simulink model "quest3"  (R2015a)
settings: Solver=ode5  StartTime=0.0  StopTime=20  FixedStep=0.001  RelTol=1e-3
values from neighbouring files (symbols this model uses):
  a = 0.3    [dynamicInit.m]
  a_e = a    (= 0.3)    [dynamicInit.m]
  d = 0.1    [dynamicInit.m]    (also in plotVehicle.m)
  r = 0.1    [dynamicInit.m]
  r_e = r    (= 0.1)    [dynamicInit.m]
undefined symbols (not defined in the file or in its folder): F_invW_1
libraries: simulink x2
settings Model: CovModelRefEnable=off  Creator=Subodh  LastModifiedBy=smishra
settings SolverCC: AlgebraicLoopSolver=LineSearch
settings DataIOCC: SaveFormat=Dataset
settings HardwareCC: ProdBitPerPointer=64  ProdLargestAtomicFloat=Float  ProdIntDivRoundTo=Zero  ProdEndianess=LittleEndian  ProdHWDeviceType=Specified
settings GRTTargetCC: GeneratePreprocessorConditionals=Use local settings

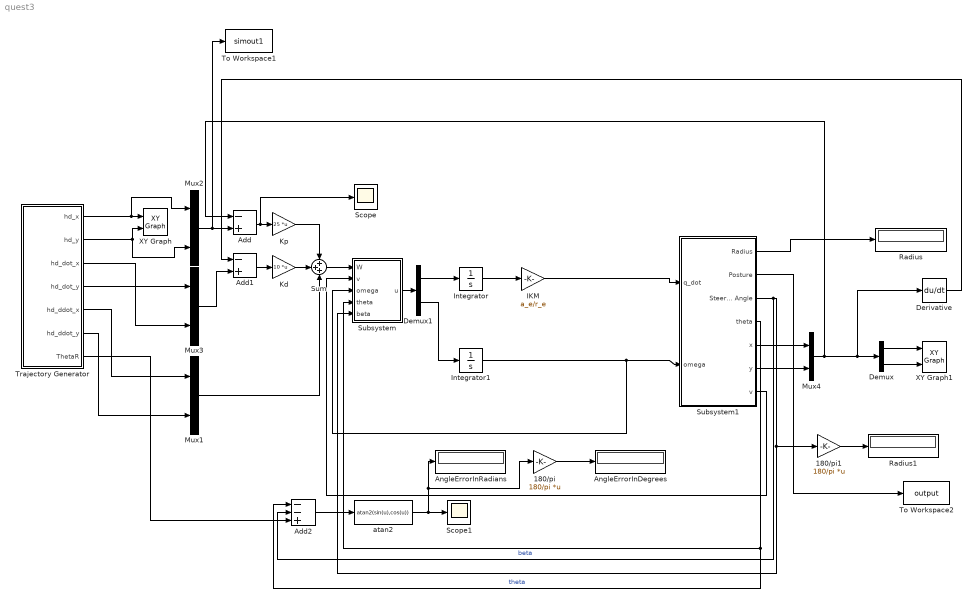
== system quest3 ==
  180/pi : Gain  Gain=180/pi  Multiplication=Matrix(K*u)
  180/pi1 : Gain  Gain=180/pi  Multiplication=Matrix(K*u)
  Add : Sum  Inputs=-+
  Add1 : Sum  Inputs=-+
  Add2 : Sum  Inputs=--+
  AngleErrorInDegrees : Display
  AngleErrorInRadians : Display
  Demux : Demux  Outputs=2
  Demux1 : Demux  Outputs=2
  Derivative : Derivative
  IKM : Gain  Gain=a_e/r_e
  Integrator : Integrator
  Integrator1 : Integrator
  Kd : Gain  Gain=10  Multiplication=Matrix(K*u)
  Kp : Gain  Gain=25  Multiplication=Matrix(K*u)
  Mux{1..4} (4 alike) : Mux  Inputs=2
  Radius : Display
  Radius1 : Display
  Scope : Scope
      settings: YMin=0.00055  YMax=0.001075
  Scope1 : Scope
      settings: YMin=304.4199  YMax=336.4641
  Subsystem : Subsystem
  Subsystem1 : Subsystem
  Sum : Sum  Inputs=+++
  To Workspace1 : ToWorkspace  VariableName=simout1  SampleTime=-1
  To Workspace2 : ToWorkspace  VariableName=output  SampleTime=-1
  Trajectory Generator : Subsystem
  XY Graph : simulink/Sinks/XY Graph  xmin=-2.3  xmax=2.3  ymin=-2.3  ymax=2.3  st=-1
  XY Graph1 : simulink/Sinks/XY Graph  xmin=-2  xmax=2  ymin=-2  ymax=2  st=-1
  atan2 : Fcn  Expr=atan2(sin(u),cos(u))
  wires:
  Trajectory Generator/1(hd_x) -> Mux2/1, XY Graph/1
  Trajectory Generator/2(hd_y) -> Mux2/2, XY Graph/2
  Trajectory Generator/3(hd_dot_x) -> Mux3/1
  Trajectory Generator/4(hd_dot_y) -> Mux3/2
  Mux2/1 -> To Workspace1/1, Add/2
  Add/1 -> Scope/1, Kp/1
  Kp/1 -> Sum/1
  Sum/1 -> Subsystem/1(W)
  Trajectory Generator/5(hd_ddot_x) -> Mux1/1
  Trajectory Generator/6(hd_ddot_y) -> Mux1/2
  Mux1/1 -> Sum/3
  Kd/1 -> Sum/2
  Add1/1 -> Kd/1
  Mux3/1 -> Add1/2
  Subsystem/1(u) -> Demux1/1
  Add2/1 -> atan2/1
  atan2/1 -> 180/pi/1, AngleErrorInRadians/1, Scope1/1
  180/pi/1 -> AngleErrorInDegrees/1
  Demux1/1 -> Integrator/1
  Integrator/1 -> IKM/1
  IKM/1 -> Subsystem1/1(q_dot)
  Demux1/2 -> Integrator1/1
  Integrator1/1 -> Subsystem/3(omega), Subsystem1/2(omega)
  Subsystem1/7(v) -> Subsystem/2(v)
  Subsystem1/4(theta) -> Add2/1, Subsystem/4(theta)  "theta"
  Subsystem1/3(Steering Angle) -> Add2/2, 180/pi1/1, Subsystem/5(beta)  "beta"
  Subsystem1/5(x) -> Mux4/1
  Subsystem1/6(y) -> Mux4/2
  Mux4/1 -> Derivative/1, Demux/1, Add/1
  Demux/1 -> XY Graph1/1
  Demux/2 -> XY Graph1/2
  Derivative/1 -> Add1/1
  Subsystem1/1("Radius ") -> Radius/1
  Subsystem1/2(Posture) -> To Workspace2/1
  180/pi1/1 -> Radius1/1
  Trajectory Generator/7(ThetaR) -> Add2/3

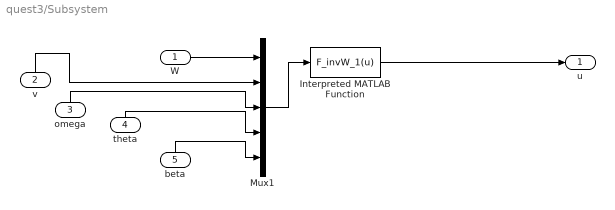
== system quest3/Subsystem ==
  W : Inport
  v : Inport  Port=2
  omega : Inport  Port=3
  theta : Inport  Port=4
  beta : Inport  Port=5
  Interpreted MATLAB Function : MATLABFcn  MATLABFcn=F_invW_1(u)  OutputDimensions=[2 1]  OutputSignalType=real  Output1D=off
  Mux1 : Mux  Inputs=5
  u : Outport
  wires:
  W/1 -> Mux1/1
  Interpreted MATLAB Function/1 -> u/1
  Mux1/1 -> Interpreted MATLAB Function/1
  omega/1 -> Mux1/3
  v/1 -> Mux1/2
  theta/1 -> Mux1/4
  beta/1 -> Mux1/5

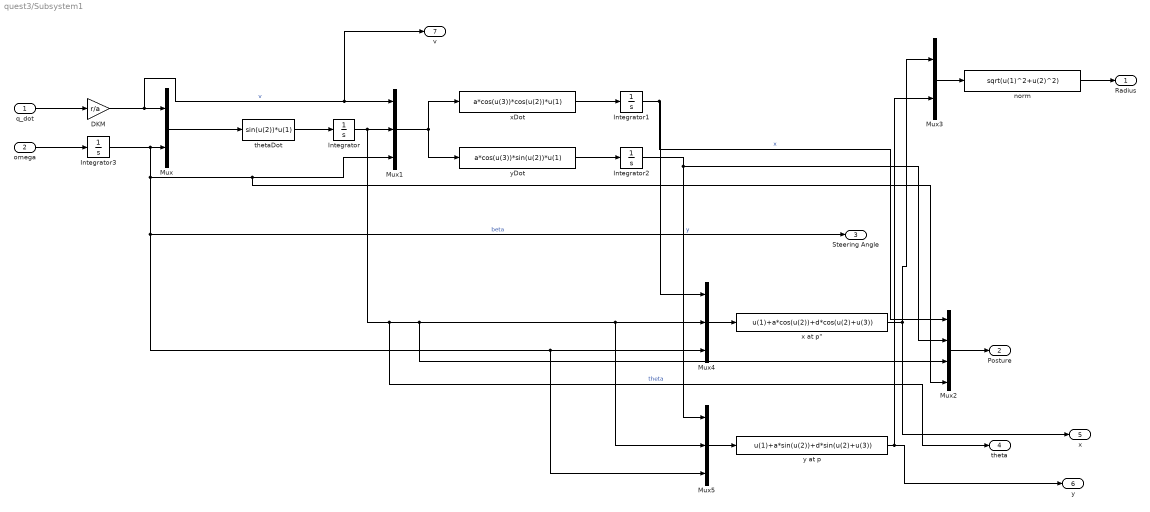
== system quest3/Subsystem1 ==
  q_dot : Inport
  omega : Inport  Port=2
  DKM : Gain  Gain=r/a
  Integrator : Integrator  InitialCondition=pi
  Integrator1 : Integrator  InitialCondition=2.3
  Integrator2 : Integrator
  Integrator3 : Integrator
  Mux : Mux  Inputs=2
  Mux1 : Mux  Inputs=3
  Mux2 : Mux
  Mux3 : Mux  Inputs=2
  Mux4 : Mux  Inputs=3
  Mux5 : Mux  Inputs=3
  norm : Fcn  Expr=sqrt(u(1)^2+u(2)^2)
  thetaDot : Fcn  Expr=sin(u(2))*u(1)
  "x at p\"" : Fcn  Expr=u(1)+a*cos(u(2))+d*cos(u(2)+u(3))
  xDot : Fcn  Expr=a*cos(u(3))*cos(u(2))*u(1)
  y at p : Fcn  Expr=u(1)+a*sin(u(2))+d*sin(u(2)+u(3))
  yDot : Fcn  Expr=a*cos(u(3))*sin(u(2))*u(1)
  "Radius " : Outport
  Posture : Outport  Port=2
  Steering Angle : Outport  Port=3
  theta : Outport  Port=4
  x : Outport  Port=5
  y : Outport  Port=6
  v : Outport  Port=7
  wires:
  Mux/1 -> thetaDot/1
  Integrator/1 -> theta/1, Mux2/3, Mux5/2, Mux4/2, Mux1/2  "theta"
  xDot/1 -> Integrator1/1
  Mux3/1 -> norm/1
  thetaDot/1 -> Integrator/1
  Mux1/1 -> xDot/1, yDot/1
  yDot/1 -> Integrator2/1
  Integrator1/1 -> Mux2/1, Mux4/1  "x"
  Integrator2/1 -> Mux2/2, Mux5/1  "y"
  Integrator3/1 -> Mux5/3, Mux4/3, Steering Angle/1, Mux2/4, Mux1/3, Mux/2  "beta"
  norm/1 -> "Radius "/1
  q_dot/1 -> DKM/1
  DKM/1 -> v/1, Mux1/1, Mux/1  "v"
  Mux4/1 -> "x at p\""/1
  Mux5/1 -> y at p/1
  "x at p\""/1 -> x/1, Mux3/1
  y at p/1 -> Mux3/2, y/1
  Mux2/1 -> Posture/1
  omega/1 -> Integrator3/1

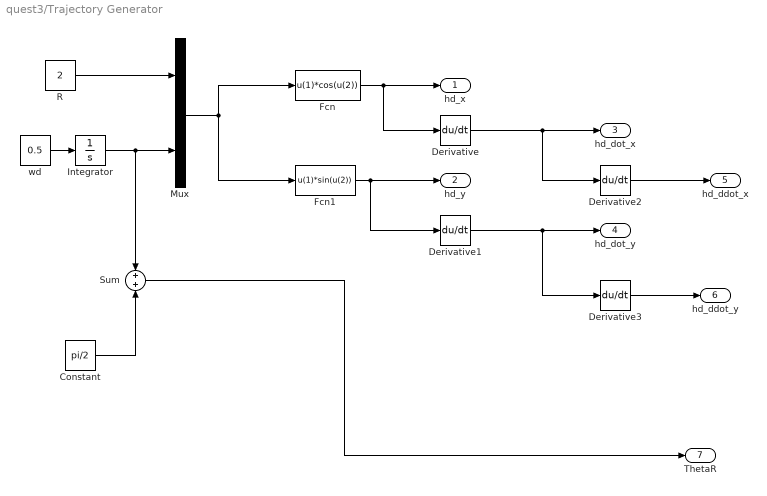
== system quest3/Trajectory Generator ==
  Constant : Constant  Value=pi/2
  Derivative{,1..3} (4 alike) : Derivative
  Fcn : Fcn  Expr=u(1)*cos(u(2))
  Fcn1 : Fcn  Expr=u(1)*sin(u(2))
  Integrator : Integrator
  Mux : Mux  Inputs=2
  R : Constant  Value=2
  Sum : Sum
  wd : Constant  Value=0.5
  hd_x : Outport
  hd_y : Outport  Port=2
  hd_dot_x : Outport  Port=3
  hd_dot_y : Outport  Port=4
  hd_ddot_x : Outport  Port=5
  hd_ddot_y : Outport  Port=6
  ThetaR : Outport  Port=7
  wires:
  Fcn/1 -> Derivative/1, hd_x/1
  Fcn1/1 -> Derivative1/1, hd_y/1
  Mux/1 -> Fcn1/1, Fcn/1
  R/1 -> Mux/1
  wd/1 -> Integrator/1
  Derivative/1 -> Derivative2/1, hd_dot_x/1
  Derivative1/1 -> Derivative3/1, hd_dot_y/1
  Derivative2/1 -> hd_ddot_x/1
  Derivative3/1 -> hd_ddot_y/1
  Constant/1 -> Sum/2
  Integrator/1 -> Sum/1, Mux/2
  Sum/1 -> ThetaR/1
